simulink model "forceControl"  (R2022b)
settings: Solver=VariableStepAuto  StartTime=0.0  StopTime=100.0  RelTol=1e-3
values from neighbouring files (symbols this model uses):
  a_1 = 1    [parameters.m]
  a_2 = 1    [parameters.m]
  kf_1 = 0.05    [parameters.m]
  kf_2 = 0.05    [parameters.m]
  kp_1 = 2500*100    (= 250000)    [parameters.m]
  kp_2 = 2500*100    (= 250000)    [parameters.m]
  md_1 = 100*1000    (= 100000)    [parameters.m]
  md_2 = 100*1000    (= 100000)    [parameters.m]
libraries: matrix_library x1
settings Model: Creator=eleves  LastModifiedBy=eleves

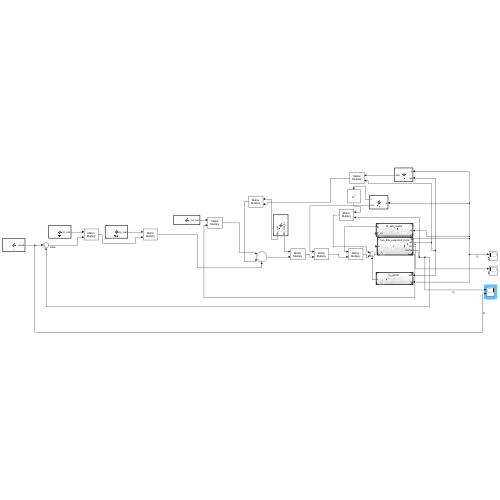
[thumbnail: Simulink's stored preview of the top-level diagram]
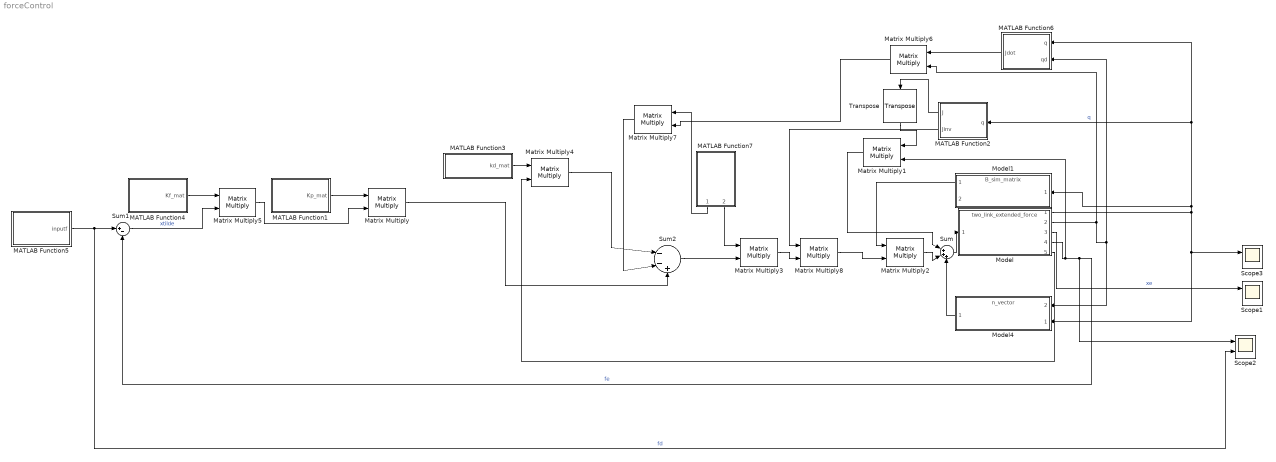
== system forceControl ==
  MATLAB Function1 : MATLAB Function  TreatAsAtomicUnit=on
  MATLAB Function2 : MATLAB Function  TreatAsAtomicUnit=on
  MATLAB Function3 : MATLAB Function  TreatAsAtomicUnit=on
  MATLAB Function4 : MATLAB Function  TreatAsAtomicUnit=on
  MATLAB Function5 : MATLAB Function  TreatAsAtomicUnit=on
  MATLAB Function6 : MATLAB Function  TreatAsAtomicUnit=on
  MATLAB Function7 : MATLAB Function  TreatAsAtomicUnit=on
  Matrix Multiply{,1..8} (9 alike) : Product  Multiplication=Matrix(*)
  Model : ModelReference  ModelNameDialog=two_link_extended_force.slx  SimulationMode=Normal  ModelReferenceVersion=1.4
  Model1 : ModelReference  ModelNameDialog=B_sim_matrix.slx  SimulationMode=Normal  ModelReferenceVersion=13.0
  Model4 : ModelReference  ModelNameDialog=n_vector.slx  SimulationMode=Normal  ModelReferenceVersion=1.3
      settings: PortSchema="{\"entries\":[{\"content\":{\"sides\":[{\"content\":{\"connectorIds\":[\"In2\",\"In1\"]},\"type\":\"ConnectorPlacement.EquallySpacedRectSide\",\"uuid\":\"0004a852-6b57-412e-a247-f7a948c02aef\"},{\"content\":{\"connectorIds\":[\"Out1\"],\"side\":\"RIGHT\"},\"type\":\"ConnectorPlacement.EquallySpacedRectSide\",\"uuid\":\"2c6a1f56-b264-4a50-8175-f4e8d5862eda\"},{\"content\":{\"connectorIds\":[],\"side\":\"TOP\"},\"type\":\"ConnectorPlacement.EquallySpacedRectSide\",\"uuid\":\"b3451316-5974-4a81-98c7-74555a3ec881\"}]},\"type\":\"ConnectorPlacement.EquallySpacedConnector\",\"uuid\":\"ac2390f0-df41-4187-a0e3-0c9a5394d303\"}],\"packageUris\":[\"http://schema.mathworks.com/mf0/Connector/R2020b\"],\"version\":\"1.0\"}"
  Scope1 : Scope  NumInputPorts=2
  Scope2 : Scope  NumInputPorts=2
  Scope3 : Scope  NumInputPorts=2
  Sum : Sum  Inputs=|+++
  Sum1 : Sum  Inputs=|+-
  Sum2 : Sum  Inputs=|--+
  Transpose : matrix_library/Transpose
  wires:
  Model/1 -> Scope3/1, Model4/1, Model1/1, MATLAB Function2/1(q), MATLAB Function6/1(q)  "q"
  Model/3 -> Scope1/1  "xe"
  Sum/1 -> Model/1
  MATLAB Function7/2(Md_mat_inv) -> Matrix Multiply3/1
  MATLAB Function6/1(Jdot) -> Matrix Multiply6/1
  Matrix Multiply6/1 -> Matrix Multiply7/2
  MATLAB Function7/1(Md_mat) -> Matrix Multiply7/1
  Matrix Multiply7/1 -> Sum2/2
  Sum2/1 -> Matrix Multiply3/2
  Model4/1 -> Sum/3
  MATLAB Function1/1(Kp_mat) -> Matrix Multiply/1
  Matrix Multiply2/1 -> Sum/2
  Model1/1 -> Matrix Multiply2/1
  Model/2 -> Model4/2, MATLAB Function6/2(qd), Matrix Multiply6/2
  Matrix Multiply8/1 -> Matrix Multiply2/2
  MATLAB Function2/1(J) -> Transpose/1
  Transpose/1 -> Matrix Multiply1/1
  Matrix Multiply1/1 -> Sum/1
  Matrix Multiply3/1 -> Matrix Multiply8/2
  MATLAB Function2/2(Jinv) -> Matrix Multiply8/1
  MATLAB Function3/1(kd_mat) -> Matrix Multiply4/1
  Matrix Multiply4/1 -> Sum2/1
  MATLAB Function4/1(Kf_mat) -> Matrix Multiply5/1
  Sum1/1 -> Matrix Multiply5/2  "xtilde"
  Model/4 -> Scope2/1, Sum1/2, Matrix Multiply1/2  "fe"
  MATLAB Function5/1(inputf) -> Scope2/2, Sum1/1  "fd"
  Matrix Multiply5/1 -> Matrix Multiply/2
  Matrix Multiply/1 -> Sum2/3
  Model/5 -> Matrix Multiply4/2

== matlab function forceControl/MATLAB Function1 ==
  data: Kp_mat output; kp_1 parameter; kp_2 parameter
function Kp_mat = fcn(kp_1, kp_2)
    Kp_mat = [kp_1,0;
              0,kp_2];
end

== matlab function forceControl/MATLAB Function4 ==
  data: Kf_mat output; kf_1 parameter; kf_2 parameter
function Kf_mat = fcn(kf_1, kf_2)
    Kf_mat = [kf_1,0;
              0,kf_2];
end

== matlab function forceControl/MATLAB Function2 ==
  data: q input; J output; a_1 parameter; a_2 parameter; Jinv output
function [J,Jinv] = fcn(q,a_1, a_2)
    theta1 = q(1);
    theta2 = q(2);
    J = [-a_1*sin(theta1)-a_2*sin(theta1+theta2),-a_2*sin(theta1+theta2);
        a_1*cos(theta1)+a_2*cos(theta1+theta2),a_2*cos(theta1+theta2)];
    Jinv = pinv(J);

end

== matlab function forceControl/MATLAB Function3 ==
  data: kd_mat output; kp_1 parameter; kp_2 parameter
function kd_mat = fcn(kp_1, kp_2)
    kd_mat = [kp_1,0;
              0,kp_2];
end

== matlab function forceControl/MATLAB Function5 ==
  data: inputf output; f_target parameter
function inputf = fcn(f_target)
    inputf = f_target;
end

== matlab function forceControl/MATLAB Function6 ==
  data: q input; qd input; Jdot output; a_1 parameter; a_2 parameter
function Jdot = fcn(q,qd,a_1, a_2)
    theta1 = q(1);
    theta2 = q(2);
    theta1d = qd(1);
    theta2d = qd(2);
    Jdot = [-a_1*theta1d*cos(theta1)-a_2*(theta1d+theta2d)*cos(theta1+theta2),-a_2*(theta1d+theta2d)*cos(theta1+theta2);
        -a_1*theta1d*sin(theta1)-a_2*(theta1d+theta2d)*sin(theta1+theta2),-a_2*(theta1d+theta2d)*sin(theta1+theta2)];

end

== matlab function forceControl/MATLAB Function7 ==
  data: Md_mat output; md_1 parameter; md_2 parameter; Md_mat_inv output
function [Md_mat,Md_mat_inv] = fcn(md_1, md_2)
    Md_mat = [md_1,0;
              0,md_2];
    Md_mat_inv = inv(Md_mat);
end
